simulink model "Task4_mdl"  (R2021a)
settings: Solver=VariableStepAuto  StartTime=0.0  StopTime=1000  RelTol=1e-3
settings Model: Creator=emiwi425  LastModifiedBy=emiwi425

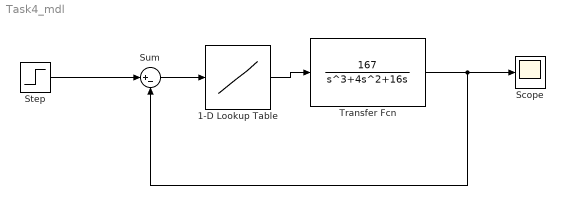
== system Task4_mdl ==
  1-D Lookup Table : Lookup_n-D  NumberOfTableDimensions=1  BreakpointsForDimension1=[-1 0 1]  Table=[-0.2 0 1]  InternalRulePriority=Speed  RndMeth=Simplest  InputSameDT=on
  Scope : Scope
  Step : Step  After=0.1  SampleTime=0
  Sum : Sum  Inputs=|+-
  Transfer Fcn : TransferFcn  Numerator=[167]  Denominator=[1 4 16 0]
  wires:
  Sum/1 -> 1-D Lookup Table/1
  Step/1 -> Sum/1
  1-D Lookup Table/1 -> Transfer Fcn/1
  Transfer Fcn/1 -> Sum/2, Scope/1
